simulink model "six_plus_six_AcmsteeringV09_main_1lf"  (R2014a)
settings: Solver=FixedStepDiscrete  StartTime=0.0  StopTime=10.0  FixedStep=0.0005  RelTol=1e-3
InitFcn:
  | Veh_Par_wxt
undefined symbols (not defined in the file or in its folder): acc_spdctl, ag_thr, B, bra_em, bra_pre_gz2, bra_pre_gz34, bra_pre_yd, brakepre_dem_data, brakeTrq_dem_data, bratrq_max, ecucoder_acal, eff_tran, ESP_switch, G, guzhang_lf, guzhang_lm, guzhang_lr, guzhang_rf, guzhang_rm, guzhang_rr, kd1, kd2, ki1, ki2, kp1, kp2, L, myFIS, premax, Radius, RC_switch, s_opt_yi, s_opt_zhuan, s_opt_zhuan_add, s_opt_zhuan_table, spd_map_mot, spd_spdctl, speed_thr_park, TCS_switch, tras_ratio, trq_map_mot, trqmax_yd, trqmax_zx, trqmaxneg, v_gain, v_table, v_thr_park, zhidong_bianmazhi, zhidong_down, zhidong_up, zhidong_youmen, zhuanxiang_bianmazhi, zhuanxiang_down, zhuanxiang_up, zhuanxiang_youmen
libraries: simulink x980, ec5744lib x59, fuzblock x2
(part 3 of 25)

== system six_plus_six_AcmsteeringV09_main_1lf/Data_input/MCU2_1 ==
  In1 : Inport
  In2 : Inport  Port=2
  Trigger : TriggerPort  TriggerType=function-call  PortDimensions=1
  MCU2 : Subsystem
  MCU2_MotorStallingFault : Outport
  MCU2_UdcDetectionFault : Outport  Port=2
  MCU2_TempSensorFault : Outport  Port=3
  MCU2_ActiveDischargingFault : Outport  Port=4
  MCU2_ldcSensorFault : Outport  Port=5
  MCU2_luSensorFault : Outport  Port=6
  MCU2_lvSensorFault : Outport  Port=7
  MCU2_FaultLevel : Outport  Port=8
  MCU2_Controllerload : Outport  Port=9
  MCU2_CanCommunicationFault : Outport  Port=10
  MCU2_MemoryFault : Outport  Port=11
  MCU2_DownratingFault : Outport  Port=12
  MCU2_IGBTFault : Outport  Port=13
  MCU2_MotorOverTemp : Outport  Port=14
  MCU2_ControllerOverTemp : Outport  Port=15
  MCU2_MotorOverSpeed : Outport  Port=16
  MCU2_RotaryInverterFault : Outport  Port=17
  MCU2_UnderVoltage : Outport  Port=18
  MCU2_OverVoltage : Outport  Port=19
  MCU2_MotorOverLoad : Outport  Port=20
  wires:
  MCU2/1(MCU2_MotorStallingFault_Out) -> MCU2_MotorStallingFault/1
  MCU2/7(MCU2_IvSensorFault_Out) -> MCU2_lvSensorFault/1
  MCU2/4(MCU2_ActieDischargingFault_Out) -> MCU2_ActiveDischargingFault/1
  MCU2/12(MCU2_DownratingFault_Out) -> MCU2_DownratingFault/1
  MCU2/13(MCU2_IGBTFault_Out) -> MCU2_IGBTFault/1
  MCU2/3(MCU2_TempSensorFault_Out) -> MCU2_TempSensorFault/1
  MCU2/10(MCU2_CanCommunicationFault_Out) -> MCU2_CanCommunicationFault/1
  MCU2/11(MCU2_MemoryFault_Out) -> MCU2_MemoryFault/1
  MCU2/14(MCU2_MotorOverTemp_Out) -> MCU2_MotorOverTemp/1
  MCU2/2(MCU2_UdcDetectionFault_Out) -> MCU2_UdcDetectionFault/1
  MCU2/5(MCU2_IdcSensorFault_Out) -> MCU2_ldcSensorFault/1
  In2/1 -> MCU2/1(input)
  In1/1 -> MCU2/Enable
  MCU2/6(MCU2_IuSensorFault_Out) -> MCU2_luSensorFault/1
  MCU2/8(MCU2_FaultLevel_Out) -> MCU2_FaultLevel/1
  MCU2/9(MCU2_ControllerOverload_Out) -> MCU2_Controllerload/1
  MCU2/20(MCU2_MotorOverLoad_Out) -> MCU2_MotorOverLoad/1
  MCU2/18(MCU2_UnderVoltage_Out) -> MCU2_UnderVoltage/1
  MCU2/19(MCU2_OverVoltage_Out) -> MCU2_OverVoltage/1
  MCU2/15(MCU2_ControllerOverTemp_Out) -> MCU2_ControllerOverTemp/1
  MCU2/16(MCU2_MotorOverSpeed_Out) -> MCU2_MotorOverSpeed/1
  MCU2/17(MCU2_RotaryInverterFault_Out) -> MCU2_RotaryInverterFault/1

== matlab function six_plus_six_AcmsteeringV09_main_1lf/MainControl/mode_control/backward/backward/Drive/驱动防滑控制TCS/直行TCS/直行/MATLAB Function5 ==
  data: TCS_switch input; flag_lf1 output; flag_lm1 output; flag_lf input; flag_lm input; flag_lr input; flag_lr1 output; flag_rf input; flag_rm input; flag_rr input; flag_rf1 output; flag_rm1 output; flag_rr1 output
 function [flag_lf1,flag_lm1,flag_lr1,flag_rf1,flag_rm1,flag_rr1] = fcn(TCS_switch,flag_lf,flag_lm,flag_lr,flag_rf,flag_rm,flag_rr)
%#codegen
if TCS_switch==0
    flag_lf1=single(0);
    flag_lm1=single(0);
    flag_lr1=single(0);
    flag_rf1=single(0);
    flag_rm1=single(0);
    flag_rr1=single(0);
else
    flag_lf1=single(flag_lf);
    flag_lm1=single(flag_lm);
    flag_lr1=single(flag_lr);
    flag_rf1=single(flag_rf);
    flag_rm1=single(flag_rm);
    flag_rr1=single(flag_rr);
end
end

== matlab function six_plus_six_AcmsteeringV09_main_1lf/Data_input/6/Enabled Subsystem/MATLAB Function1 ==
  data: data1 input; y output; data2 input; data3 input; data4 input
function y = fcn(data1,data2,data3,data4)
%#codegen
y1=data4*256^3+data3*256^2+data2*256+data1;
y=typecast(uint32(y1),'single');
end
% y = u;

== matlab function six_plus_six_AcmsteeringV09_main_1lf/Data_input/10/Enabled Subsystem/MATLAB Function ==
  data: data1 input; y output; data2 input; data3 input; data4 input
function y = fcn(data1,data2,data3,data4)
%#codegen
y1=data4*256^3+data3*256^2+data2*256+data1;
y=typecast(uint32(y1),'single');
end
% y = u;

== matlab function six_plus_six_AcmsteeringV09_main_1lf/MainControl/mode_control/backward/backward/Drive/MATLAB Function ==
  data: acc_y input; y output; ag_thr input
function y = fcn(acc_y,ag_thr)
%#codegen
if abs(acc_y)>=ag_thr
    y=int8(0);
else 
    y=int8(1);
end
end

== system six_plus_six_AcmsteeringV09_main_1lf/Data_input/MCU2_2 ==
  In1 : Inport
  In2 : Inport  Port=2
  Trigger : TriggerPort  TriggerType=function-call  PortDimensions=1
  MCU2 : Subsystem
  MCU2_MotorStallingFault : Outport
  MCU2_UdcDetectionFault : Outport  Port=2
  MCU2_TempSensorFault : Outport  Port=3
  MCU2_ActiveDischargingFault : Outport  Port=4
  MCU2_ldcSensorFault : Outport  Port=5
  MCU2_luSensorFault : Outport  Port=6
  MCU2_lvSensorFault : Outport  Port=7
  MCU2_FaultLevel : Outport  Port=8
  MCU2_Controllerload : Outport  Port=9
  MCU2_CanCommunicationFault : Outport  Port=10
  MCU2_MemoryFault : Outport  Port=11
  MCU2_DownratingFault : Outport  Port=12
  MCU2_IGBTFault : Outport  Port=13
  MCU2_MotorOverTemp : Outport  Port=14
  MCU2_ControllerOverTemp : Outport  Port=15
  MCU2_MotorOverSpeed : Outport  Port=16
  MCU2_RotaryInverterFault : Outport  Port=17
  MCU2_UnderVoltage : Outport  Port=18
  MCU2_OverVoltage : Outport  Port=19
  MCU2_MotorOverLoad : Outport  Port=20
  wires:
  MCU2/1(MCU2_MotorStallingFault_Out) -> MCU2_MotorStallingFault/1
  MCU2/7(MCU2_IvSensorFault_Out) -> MCU2_lvSensorFault/1
  MCU2/4(MCU2_ActieDischargingFault_Out) -> MCU2_ActiveDischargingFault/1
  MCU2/12(MCU2_DownratingFault_Out) -> MCU2_DownratingFault/1
  MCU2/13(MCU2_IGBTFault_Out) -> MCU2_IGBTFault/1
  MCU2/3(MCU2_TempSensorFault_Out) -> MCU2_TempSensorFault/1
  MCU2/10(MCU2_CanCommunicationFault_Out) -> MCU2_CanCommunicationFault/1
  MCU2/11(MCU2_MemoryFault_Out) -> MCU2_MemoryFault/1
  MCU2/14(MCU2_MotorOverTemp_Out) -> MCU2_MotorOverTemp/1
  MCU2/2(MCU2_UdcDetectionFault_Out) -> MCU2_UdcDetectionFault/1
  MCU2/5(MCU2_IdcSensorFault_Out) -> MCU2_ldcSensorFault/1
  In2/1 -> MCU2/1(input)
  In1/1 -> MCU2/Enable
  MCU2/6(MCU2_IuSensorFault_Out) -> MCU2_luSensorFault/1
  MCU2/8(MCU2_FaultLevel_Out) -> MCU2_FaultLevel/1
  MCU2/9(MCU2_ControllerOverload_Out) -> MCU2_Controllerload/1
  MCU2/20(MCU2_MotorOverLoad_Out) -> MCU2_MotorOverLoad/1
  MCU2/18(MCU2_UnderVoltage_Out) -> MCU2_UnderVoltage/1
  MCU2/19(MCU2_OverVoltage_Out) -> MCU2_OverVoltage/1
  MCU2/15(MCU2_ControllerOverTemp_Out) -> MCU2_ControllerOverTemp/1
  MCU2/16(MCU2_MotorOverSpeed_Out) -> MCU2_MotorOverSpeed/1
  MCU2/17(MCU2_RotaryInverterFault_Out) -> MCU2_RotaryInverterFault/1

== system six_plus_six_AcmsteeringV09_main_1lf/Data_input/MCU2_3 ==
  In1 : Inport
  In2 : Inport  Port=2
  Trigger : TriggerPort  TriggerType=function-call  PortDimensions=1
  MCU2 : Subsystem
  MCU2_MotorStallingFault : Outport
  MCU2_UdcDetectionFault : Outport  Port=2
  MCU2_TempSensorFault : Outport  Port=3
  MCU2_ActiveDischargingFault : Outport  Port=4
  MCU2_ldcSensorFault : Outport  Port=5
  MCU2_luSensorFault : Outport  Port=6
  MCU2_lvSensorFault : Outport  Port=7
  MCU2_FaultLevel : Outport  Port=8
  MCU2_Controllerload : Outport  Port=9
  MCU2_CanCommunicationFault : Outport  Port=10
  MCU2_MemoryFault : Outport  Port=11
  MCU2_DownratingFault : Outport  Port=12
  MCU2_IGBTFault : Outport  Port=13
  MCU2_MotorOverTemp : Outport  Port=14
  MCU2_ControllerOverTemp : Outport  Port=15
  MCU2_MotorOverSpeed : Outport  Port=16
  MCU2_RotaryInverterFault : Outport  Port=17
  MCU2_UnderVoltage : Outport  Port=18
  MCU2_OverVoltage : Outport  Port=19
  MCU2_MotorOverLoad : Outport  Port=20
  wires:
  MCU2/1(MCU2_MotorStallingFault_Out) -> MCU2_MotorStallingFault/1
  MCU2/7(MCU2_IvSensorFault_Out) -> MCU2_lvSensorFault/1
  MCU2/4(MCU2_ActieDischargingFault_Out) -> MCU2_ActiveDischargingFault/1
  MCU2/12(MCU2_DownratingFault_Out) -> MCU2_DownratingFault/1
  MCU2/13(MCU2_IGBTFault_Out) -> MCU2_IGBTFault/1
  MCU2/3(MCU2_TempSensorFault_Out) -> MCU2_TempSensorFault/1
  MCU2/10(MCU2_CanCommunicationFault_Out) -> MCU2_CanCommunicationFault/1
  MCU2/11(MCU2_MemoryFault_Out) -> MCU2_MemoryFault/1
  MCU2/14(MCU2_MotorOverTemp_Out) -> MCU2_MotorOverTemp/1
  MCU2/2(MCU2_UdcDetectionFault_Out) -> MCU2_UdcDetectionFault/1
  MCU2/5(MCU2_IdcSensorFault_Out) -> MCU2_ldcSensorFault/1
  In2/1 -> MCU2/1(input)
  In1/1 -> MCU2/Enable
  MCU2/6(MCU2_IuSensorFault_Out) -> MCU2_luSensorFault/1
  MCU2/8(MCU2_FaultLevel_Out) -> MCU2_FaultLevel/1
  MCU2/9(MCU2_ControllerOverload_Out) -> MCU2_Controllerload/1
  MCU2/20(MCU2_MotorOverLoad_Out) -> MCU2_MotorOverLoad/1
  MCU2/18(MCU2_UnderVoltage_Out) -> MCU2_UnderVoltage/1
  MCU2/19(MCU2_OverVoltage_Out) -> MCU2_OverVoltage/1
  MCU2/15(MCU2_ControllerOverTemp_Out) -> MCU2_ControllerOverTemp/1
  MCU2/16(MCU2_MotorOverSpeed_Out) -> MCU2_MotorOverSpeed/1
  MCU2/17(MCU2_RotaryInverterFault_Out) -> MCU2_RotaryInverterFault/1

== system six_plus_six_AcmsteeringV09_main_1lf/Data_input/MCU2_4 ==
  In1 : Inport
  In2 : Inport  Port=2
  Trigger : TriggerPort  TriggerType=function-call  PortDimensions=1
  MCU2 : Subsystem
  MCU2_MotorStallingFault : Outport
  MCU2_UdcDetectionFault : Outport  Port=2
  MCU2_TempSensorFault : Outport  Port=3
  MCU2_ActiveDischargingFault : Outport  Port=4
  MCU2_ldcSensorFault : Outport  Port=5
  MCU2_luSensorFault : Outport  Port=6
  MCU2_lvSensorFault : Outport  Port=7
  MCU2_FaultLevel : Outport  Port=8
  MCU2_Controllerload : Outport  Port=9
  MCU2_CanCommunicationFault : Outport  Port=10
  MCU2_MemoryFault : Outport  Port=11
  MCU2_DownratingFault : Outport  Port=12
  MCU2_IGBTFault : Outport  Port=13
  MCU2_MotorOverTemp : Outport  Port=14
  MCU2_ControllerOverTemp : Outport  Port=15
  MCU2_MotorOverSpeed : Outport  Port=16
  MCU2_RotaryInverterFault : Outport  Port=17
  MCU2_UnderVoltage : Outport  Port=18
  MCU2_OverVoltage : Outport  Port=19
  MCU2_MotorOverLoad : Outport  Port=20
  wires:
  MCU2/1(MCU2_MotorStallingFault_Out) -> MCU2_MotorStallingFault/1
  MCU2/7(MCU2_IvSensorFault_Out) -> MCU2_lvSensorFault/1
  MCU2/4(MCU2_ActieDischargingFault_Out) -> MCU2_ActiveDischargingFault/1
  MCU2/12(MCU2_DownratingFault_Out) -> MCU2_DownratingFault/1
  MCU2/13(MCU2_IGBTFault_Out) -> MCU2_IGBTFault/1
  MCU2/3(MCU2_TempSensorFault_Out) -> MCU2_TempSensorFault/1
  MCU2/10(MCU2_CanCommunicationFault_Out) -> MCU2_CanCommunicationFault/1
  MCU2/11(MCU2_MemoryFault_Out) -> MCU2_MemoryFault/1
  MCU2/14(MCU2_MotorOverTemp_Out) -> MCU2_MotorOverTemp/1
  MCU2/2(MCU2_UdcDetectionFault_Out) -> MCU2_UdcDetectionFault/1
  MCU2/5(MCU2_IdcSensorFault_Out) -> MCU2_ldcSensorFault/1
  In2/1 -> MCU2/1(input)
  In1/1 -> MCU2/Enable
  MCU2/6(MCU2_IuSensorFault_Out) -> MCU2_luSensorFault/1
  MCU2/8(MCU2_FaultLevel_Out) -> MCU2_FaultLevel/1
  MCU2/9(MCU2_ControllerOverload_Out) -> MCU2_Controllerload/1
  MCU2/20(MCU2_MotorOverLoad_Out) -> MCU2_MotorOverLoad/1
  MCU2/18(MCU2_UnderVoltage_Out) -> MCU2_UnderVoltage/1
  MCU2/19(MCU2_OverVoltage_Out) -> MCU2_OverVoltage/1
  MCU2/15(MCU2_ControllerOverTemp_Out) -> MCU2_ControllerOverTemp/1
  MCU2/16(MCU2_MotorOverSpeed_Out) -> MCU2_MotorOverSpeed/1
  MCU2/17(MCU2_RotaryInverterFault_Out) -> MCU2_RotaryInverterFault/1

== system six_plus_six_AcmsteeringV09_main_1lf/Data_input/MCU2_5 ==
  In1 : Inport
  In2 : Inport  Port=2
  Trigger : TriggerPort  TriggerType=function-call  PortDimensions=1
  MCU2 : Subsystem
  MCU2_MotorStallingFault : Outport
  MCU2_UdcDetectionFault : Outport  Port=2
  MCU2_TempSensorFault : Outport  Port=3
  MCU2_ActiveDischargingFault : Outport  Port=4
  MCU2_ldcSensorFault : Outport  Port=5
  MCU2_luSensorFault : Outport  Port=6
  MCU2_lvSensorFault : Outport  Port=7
  MCU2_FaultLevel : Outport  Port=8
  MCU2_Controllerload : Outport  Port=9
  MCU2_CanCommunicationFault : Outport  Port=10
  MCU2_MemoryFault : Outport  Port=11
  MCU2_DownratingFault : Outport  Port=12
  MCU2_IGBTFault : Outport  Port=13
  MCU2_MotorOverTemp : Outport  Port=14
  MCU2_ControllerOverTemp : Outport  Port=15
  MCU2_MotorOverSpeed : Outport  Port=16
  MCU2_RotaryInverterFault : Outport  Port=17
  MCU2_UnderVoltage : Outport  Port=18
  MCU2_OverVoltage : Outport  Port=19
  MCU2_MotorOverLoad : Outport  Port=20
  wires:
  MCU2/1(MCU2_MotorStallingFault_Out) -> MCU2_MotorStallingFault/1
  MCU2/7(MCU2_IvSensorFault_Out) -> MCU2_lvSensorFault/1
  MCU2/4(MCU2_ActieDischargingFault_Out) -> MCU2_ActiveDischargingFault/1
  MCU2/12(MCU2_DownratingFault_Out) -> MCU2_DownratingFault/1
  MCU2/13(MCU2_IGBTFault_Out) -> MCU2_IGBTFault/1
  MCU2/3(MCU2_TempSensorFault_Out) -> MCU2_TempSensorFault/1
  MCU2/10(MCU2_CanCommunicationFault_Out) -> MCU2_CanCommunicationFault/1
  MCU2/11(MCU2_MemoryFault_Out) -> MCU2_MemoryFault/1
  MCU2/14(MCU2_MotorOverTemp_Out) -> MCU2_MotorOverTemp/1
  MCU2/2(MCU2_UdcDetectionFault_Out) -> MCU2_UdcDetectionFault/1
  MCU2/5(MCU2_IdcSensorFault_Out) -> MCU2_ldcSensorFault/1
  In2/1 -> MCU2/1(input)
  In1/1 -> MCU2/Enable
  MCU2/6(MCU2_IuSensorFault_Out) -> MCU2_luSensorFault/1
  MCU2/8(MCU2_FaultLevel_Out) -> MCU2_FaultLevel/1
  MCU2/9(MCU2_ControllerOverload_Out) -> MCU2_Controllerload/1
  MCU2/20(MCU2_MotorOverLoad_Out) -> MCU2_MotorOverLoad/1
  MCU2/18(MCU2_UnderVoltage_Out) -> MCU2_UnderVoltage/1
  MCU2/19(MCU2_OverVoltage_Out) -> MCU2_OverVoltage/1
  MCU2/15(MCU2_ControllerOverTemp_Out) -> MCU2_ControllerOverTemp/1
  MCU2/16(MCU2_MotorOverSpeed_Out) -> MCU2_MotorOverSpeed/1
  MCU2/17(MCU2_RotaryInverterFault_Out) -> MCU2_RotaryInverterFault/1

== system six_plus_six_AcmsteeringV09_main_1lf/Data_input/RemoteControl1 ==
  In1 : Inport
  In2 : Inport  Port=2
  Trigger : TriggerPort  TriggerType=function-call  PortDimensions=1
  Yaokong2 : Subsystem
  SH : Outport
  SE : Outport  Port=2
  SD : Outport  Port=3
  SA : Outport  Port=4
  LIFEspan : Outport  Port=5
  wires:
  Yaokong2/2(SE_Out) -> SE/1
  Yaokong2/3(SD_Out) -> SD/1
  Yaokong2/4(SA_Out) -> SA/1
  In2/1 -> Yaokong2/1(input)
  In1/1 -> Yaokong2/Enable
  Yaokong2/1(SH_Out) -> SH/1
  Yaokong2/5(LIFEspan_Out) -> LIFEspan/1

== system six_plus_six_AcmsteeringV09_main_1lf/Data_input/RemoteControl2 ==
  In1 : Inport
  In2 : Inport  Port=2
  Trigger : TriggerPort  TriggerType=function-call  PortDimensions=1
  Yaokong1 : Subsystem
  Rightstick_updown : Outport
  Rightstick_leftright : Outport  Port=2
  Leftstick_updown : Outport  Port=3
  Leftstick_leftright : Outport  Port=4
  wires:
  In1/1 -> Yaokong1/Enable
  In2/1 -> Yaokong1/1(input)
  Yaokong1/1(Rightstick_updown_Out) -> Rightstick_updown/1
  Yaokong1/2(Rightstick_leftright_Out) -> Rightstick_leftright/1
  Yaokong1/3(Leftstick_updown_Out) -> Leftstick_updown/1
  Yaokong1/4(Leftstick_leftright_Out) -> Leftstick_leftright/1

== system six_plus_six_AcmsteeringV09_main_1lf/MainControl/mode_control ==
  mode_dem_out : Inport
  Signals : Inport  Port=2
  Multiport Switch : MultiPortSwitch  DataPortOrder=Zero-based contiguous  Inputs=6
  Park : Subsystem  TreatAsAtomicUnit=on
  Switch Case : SwitchCase  CaseConditions={0,1,2,3,4,5}  ShowDefaultCase=off
  backward : Subsystem  TreatAsAtomicUnit=on
  center_steer : Subsystem  TreatAsAtomicUnit=on
  emergency_stop : Subsystem  TreatAsAtomicUnit=on
  forward : Subsystem  TreatAsAtomicUnit=on
  neutral : Subsystem  TreatAsAtomicUnit=on
  com_dem : Outport
  wires:
  mode_dem_out/1 -> Multiport Switch/1, Switch Case/1
  Signals/1 -> backward/1(Signals), emergency_stop/1(Signals), center_steer/1(Signals), neutral/1(Signals), forward/1(Signals), Park/1(Signals)
  Switch Case/1 -> Park/Action
  Switch Case/6 -> emergency_stop/Action
  Switch Case/5 -> center_steer/Action
  Switch Case/4 -> backward/Action
  Switch Case/3 -> neutral/Action
  Switch Case/2 -> forward/Action
  Park/1(park_dem) -> Multiport Switch/2
  forward/1(forward_dem) -> Multiport Switch/3
  backward/1(backward_dem) -> Multiport Switch/5
  neutral/1(neutral_dem) -> Multiport Switch/4
  center_steer/1(center_steer_dem) -> Multiport Switch/6
  emergency_stop/1(emergency_stop_dem) -> Multiport Switch/7
  Multiport Switch/1 -> com_dem/1

== system six_plus_six_AcmsteeringV09_main_1lf/MainControl/mode_switch ==
  Signals : Inport
  Abs{,1..5} (6 alike) : Abs  OutDataTypeStr=single
  Bus Selector : BusSelector  OutputSignals=RemoteControl_dem.brake_emerg,RemoteControl_dem.park,RemoteControl_dem.acc_dem,RemoteControl_dem.steer_dem,RemoteControl_dem.brake_dem,RemoteControl_dem.center,MOTOR.MOTOR1.MCU0.MCU0_SpeedFdk,MOTOR.MOTOR2.MCU0_1.MCU0_1SpeedFdk,MOTOR.MOTOR3.MCU0_2.MCU0_2SpeedFdk,MOTOR.MOTOR4.MCU0_3.MCU0_3SpeedFdk,MOTOR.MOTOR5.MCU0_4.MCU0_4SpeedFdk,MOTOR.MOTOR6.MCU0_5.MCU0_5SpeedFdk
  Constant1 : Constant  Value=v_thr_park  OutDataTypeStr=single  SampleTime=-1
  Constant2 : Constant  Value=speed_thr_park  OutDataTypeStr=single  SampleTime=-1
  Memory : Memory  InheritSampleTime=on
  Terminator : Terminator
  mode_switch : MATLAB Function  TreatAsAtomicUnit=on
  mode_dem_out : Outport
  wires:
  Memory/1 -> mode_switch/14(mode_dem_out_pre)
  Signals/1 -> Bus Selector/1
  Constant2/1 -> mode_switch/13(speed_thr_park)
  mode_switch/1(mode_dem_out) -> Memory/1, mode_dem_out/1  "mode_dem_out"
  Bus Selector/1 -> mode_switch/1(brake_emerg)  "<brake_emerg>"
  Bus Selector/2 -> mode_switch/2(park)  "<park>"
  Bus Selector/3 -> mode_switch/3(acc_dem)  "<acc_dem>"
  Bus Selector/4 -> mode_switch/4(steer_dem)  "<steer_dem>"
  Bus Selector/5 -> mode_switch/5(brake_dem)  "<brake_dem>"
  Bus Selector/7 -> Abs/1  "<MCU0_SpeedFdk>"
  Bus Selector/8 -> Abs1/1  "<MCU0_1SpeedFdk>"
  Bus Selector/9 -> Abs2/1  "<MCU0_2SpeedFdk>"
  Bus Selector/10 -> Abs3/1  "<MCU0_3SpeedFdk>"
  Bus Selector/11 -> Abs4/1  "<MCU0_4SpeedFdk>"
  Bus Selector/12 -> Abs5/1  "<MCU0_5SpeedFdk>"
  Abs/1 -> mode_switch/7(MCU0_SpeedFdk)
  Abs1/1 -> mode_switch/8(MCU0_1SpeedFdk)
  Abs2/1 -> mode_switch/9(MCU0_2SpeedFdk)
  Abs3/1 -> mode_switch/10(MCU0_3SpeedFdk)
  Abs4/1 -> mode_switch/11(MCU0_4SpeedFdk)
  Abs5/1 -> mode_switch/12(MCU0_5SpeedFdk)
  Constant1/1 -> Terminator/1
  Bus Selector/6 -> mode_switch/6(center)  "<center>"

== system six_plus_six_AcmsteeringV09_main_1lf/Subsystem/VCU1 ==
  VCU1_EnableReq_in : Inport
  VCU1_CtrlModel_in : Inport  Port=2
  VCU1_GearCmd_in : Inport  Port=3
  VCU1_SpeedMax_in : Inport  Port=4
  VCU1_TorqueRef_in : Inport  Port=5
  VCU1_LifeCnt_in : Inport  Port=6
  Conv{1..8} (8 alike) : DataTypeConversion
  VCU1_CtrlModel : Subsystem
  VCU1_DLC : Constant  Value=8  OutDataTypeStr=uint8
  VCU1_DLC_Out : Terminator
  VCU1_EnableReq : Subsystem
  VCU1_GearCmd : Subsystem
  VCU1_ID : Constant  Value=2353065767  OutDataTypeStr=single
  VCU1_ID_Out : Terminator
  VCU1_LifeCnt : Subsystem
  VCU1_SpeedMax : Subsystem
  VCU1_TorqueRef : Subsystem
  VCU1_mux : Mux  Inputs=8
  or{1..8} (8 alike) : simulink/Logic and Bit Operations/Bitwise Operator  logicop=OR  UseBitMask=off  NumInputPorts=6  BitMask=bin2dec('11011001')  BitMaskRealWorld=Stored Integer
  output : Outport
  wires:
  VCU1_mux/1 -> output/1
  VCU1_LifeCnt/1(output1) -> or1/1
  VCU1_LifeCnt/2(output2) -> or2/1
  VCU1_LifeCnt/3(output3) -> or3/1
  VCU1_LifeCnt/4(output4) -> or4/1
  VCU1_LifeCnt/5(output5) -> or5/1
  VCU1_LifeCnt/6(output6) -> or6/1
  VCU1_LifeCnt/7(output7) -> or7/1
  VCU1_LifeCnt/8(output8) -> or8/1
  VCU1_TorqueRef/1(output1) -> or1/2
  VCU1_TorqueRef/2(output2) -> or2/2
  VCU1_TorqueRef/3(output3) -> or3/2
  VCU1_TorqueRef/4(output4) -> or4/2
  VCU1_TorqueRef/5(output5) -> or5/2
  VCU1_TorqueRef/6(output6) -> or6/2
  VCU1_TorqueRef/7(output7) -> or7/2
  VCU1_TorqueRef/8(output8) -> or8/2
  VCU1_SpeedMax/1(output1) -> or1/3
  VCU1_SpeedMax/2(output2) -> or2/3
  VCU1_SpeedMax/3(output3) -> or3/3
  VCU1_SpeedMax/4(output4) -> or4/3
  VCU1_SpeedMax/5(output5) -> or5/3
  VCU1_SpeedMax/6(output6) -> or6/3
  VCU1_SpeedMax/7(output7) -> or7/3
  VCU1_SpeedMax/8(output8) -> or8/3
  VCU1_GearCmd/1(output1) -> or1/4
  VCU1_GearCmd/2(output2) -> or2/4
  VCU1_GearCmd/3(output3) -> or3/4
  VCU1_GearCmd/4(output4) -> or4/4
  VCU1_GearCmd/5(output5) -> or5/4
  VCU1_GearCmd/6(output6) -> or6/4
  VCU1_GearCmd/7(output7) -> or7/4
  VCU1_GearCmd/8(output8) -> or8/4
  VCU1_CtrlModel/1(output1) -> or1/5
  VCU1_CtrlModel/2(output2) -> or2/5
  VCU1_CtrlModel/3(output3) -> or3/5
  VCU1_CtrlModel/4(output4) -> or4/5
  VCU1_CtrlModel/5(output5) -> or5/5
  VCU1_CtrlModel/6(output6) -> or6/5
  VCU1_CtrlModel/7(output7) -> or7/5
  VCU1_CtrlModel/8(output8) -> or8/5
  VCU1_EnableReq/1(output1) -> or1/6
  VCU1_EnableReq/2(output2) -> or2/6
  VCU1_EnableReq/3(output3) -> or3/6
  VCU1_EnableReq/4(output4) -> or4/6
  VCU1_EnableReq/5(output5) -> or5/6
  VCU1_EnableReq/6(output6) -> or6/6
  VCU1_EnableReq/7(output7) -> or7/6
  VCU1_EnableReq/8(output8) -> or8/6
  or1/1 -> Conv1/1
  Conv1/1 -> VCU1_mux/1
  or2/1 -> Conv2/1
  Conv2/1 -> VCU1_mux/2
  or3/1 -> Conv3/1
  Conv3/1 -> VCU1_mux/3
  or4/1 -> Conv4/1
  Conv4/1 -> VCU1_mux/4
  or5/1 -> Conv5/1
  Conv5/1 -> VCU1_mux/5
  or6/1 -> Conv6/1
  Conv6/1 -> VCU1_mux/6
  or7/1 -> Conv7/1
  Conv7/1 -> VCU1_mux/7
  or8/1 -> Conv8/1
  Conv8/1 -> VCU1_mux/8
  VCU1_ID/1 -> VCU1_ID_Out/1
  VCU1_DLC/1 -> VCU1_DLC_Out/1
  VCU1_LifeCnt_in/1 -> VCU1_LifeCnt/1(VCU1_LifeCnt)
  VCU1_TorqueRef_in/1 -> VCU1_TorqueRef/1(VCU1_TorqueRef)
  VCU1_SpeedMax_in/1 -> VCU1_SpeedMax/1(VCU1_SpeedMax)
  VCU1_GearCmd_in/1 -> VCU1_GearCmd/1(VCU1_GearCmd)
  VCU1_CtrlModel_in/1 -> VCU1_CtrlModel/1(VCU1_CtrlModel)
  VCU1_EnableReq_in/1 -> VCU1_EnableReq/1(VCU1_EnableReq)

== system six_plus_six_AcmsteeringV09_main_1lf/Subsystem/VCU2 ==
  VCU1_EnableReq_in : Inport
  VCU1_CtrlModel_in : Inport  Port=2
  VCU1_GearCmd_in : Inport  Port=3
  VCU1_SpeedMax_in : Inport  Port=4
  VCU1_TorqueRef_in : Inport  Port=5
  VCU1_LifeCnt_in : Inport  Port=6
  Conv{1..8} (8 alike) : DataTypeConversion
  VCU1_CtrlModel : Subsystem
  VCU1_DLC : Constant  Value=8  OutDataTypeStr=uint8
  VCU1_DLC_Out : Terminator
  VCU1_EnableReq : Subsystem
  VCU1_GearCmd : Subsystem
  VCU1_ID : Constant  Value=2353065767  OutDataTypeStr=single
  VCU1_ID_Out : Terminator
  VCU1_LifeCnt : Subsystem
  VCU1_SpeedMax : Subsystem
  VCU1_TorqueRef : Subsystem
  VCU1_mux : Mux  Inputs=8
  or{1..8} (8 alike) : simulink/Logic and Bit Operations/Bitwise Operator  logicop=OR  UseBitMask=off  NumInputPorts=6  BitMask=bin2dec('11011001')  BitMaskRealWorld=Stored Integer
  output : Outport
  wires:
  VCU1_mux/1 -> output/1
  VCU1_LifeCnt/1(output1) -> or1/1
  VCU1_LifeCnt/2(output2) -> or2/1
  VCU1_LifeCnt/3(output3) -> or3/1
  VCU1_LifeCnt/4(output4) -> or4/1
  VCU1_LifeCnt/5(output5) -> or5/1
  VCU1_LifeCnt/6(output6) -> or6/1
  VCU1_LifeCnt/7(output7) -> or7/1
  VCU1_LifeCnt/8(output8) -> or8/1
  VCU1_TorqueRef/1(output1) -> or1/2
  VCU1_TorqueRef/2(output2) -> or2/2
  VCU1_TorqueRef/3(output3) -> or3/2
  VCU1_TorqueRef/4(output4) -> or4/2
  VCU1_TorqueRef/5(output5) -> or5/2
  VCU1_TorqueRef/6(output6) -> or6/2
  VCU1_TorqueRef/7(output7) -> or7/2
  VCU1_TorqueRef/8(output8) -> or8/2
  VCU1_SpeedMax/1(output1) -> or1/3
  VCU1_SpeedMax/2(output2) -> or2/3
  VCU1_SpeedMax/3(output3) -> or3/3
  VCU1_SpeedMax/4(output4) -> or4/3
  VCU1_SpeedMax/5(output5) -> or5/3
  VCU1_SpeedMax/6(output6) -> or6/3
  VCU1_SpeedMax/7(output7) -> or7/3
  VCU1_SpeedMax/8(output8) -> or8/3
  VCU1_GearCmd/1(output1) -> or1/4
  VCU1_GearCmd/2(output2) -> or2/4
  VCU1_GearCmd/3(output3) -> or3/4
  VCU1_GearCmd/4(output4) -> or4/4
  VCU1_GearCmd/5(output5) -> or5/4
  VCU1_GearCmd/6(output6) -> or6/4
  VCU1_GearCmd/7(output7) -> or7/4
  VCU1_GearCmd/8(output8) -> or8/4
  VCU1_CtrlModel/1(output1) -> or1/5
  VCU1_CtrlModel/2(output2) -> or2/5
  VCU1_CtrlModel/3(output3) -> or3/5
  VCU1_CtrlModel/4(output4) -> or4/5
  VCU1_CtrlModel/5(output5) -> or5/5
  VCU1_CtrlModel/6(output6) -> or6/5
  VCU1_CtrlModel/7(output7) -> or7/5
  VCU1_CtrlModel/8(output8) -> or8/5
  VCU1_EnableReq/1(output1) -> or1/6
  VCU1_EnableReq/2(output2) -> or2/6
  VCU1_EnableReq/3(output3) -> or3/6
  VCU1_EnableReq/4(output4) -> or4/6
  VCU1_EnableReq/5(output5) -> or5/6
  VCU1_EnableReq/6(output6) -> or6/6
  VCU1_EnableReq/7(output7) -> or7/6
  VCU1_EnableReq/8(output8) -> or8/6
  or1/1 -> Conv1/1
  Conv1/1 -> VCU1_mux/1
  or2/1 -> Conv2/1
  Conv2/1 -> VCU1_mux/2
  or3/1 -> Conv3/1
  Conv3/1 -> VCU1_mux/3
  or4/1 -> Conv4/1
  Conv4/1 -> VCU1_mux/4
  or5/1 -> Conv5/1
  Conv5/1 -> VCU1_mux/5
  or6/1 -> Conv6/1
  Conv6/1 -> VCU1_mux/6
  or7/1 -> Conv7/1
  Conv7/1 -> VCU1_mux/7
  or8/1 -> Conv8/1
  Conv8/1 -> VCU1_mux/8
  VCU1_ID/1 -> VCU1_ID_Out/1
  VCU1_DLC/1 -> VCU1_DLC_Out/1
  VCU1_LifeCnt_in/1 -> VCU1_LifeCnt/1(VCU1_LifeCnt)
  VCU1_TorqueRef_in/1 -> VCU1_TorqueRef/1(VCU1_TorqueRef)
  VCU1_SpeedMax_in/1 -> VCU1_SpeedMax/1(VCU1_SpeedMax)
  VCU1_GearCmd_in/1 -> VCU1_GearCmd/1(VCU1_GearCmd)
  VCU1_CtrlModel_in/1 -> VCU1_CtrlModel/1(VCU1_CtrlModel)
  VCU1_EnableReq_in/1 -> VCU1_EnableReq/1(VCU1_EnableReq)

== system six_plus_six_AcmsteeringV09_main_1lf/Subsystem/VCU3 ==
  VCU1_EnableReq_in : Inport
  VCU1_CtrlModel_in : Inport  Port=2
  VCU1_GearCmd_in : Inport  Port=3
  VCU1_SpeedMax_in : Inport  Port=4
  VCU1_TorqueRef_in : Inport  Port=5
  VCU1_LifeCnt_in : Inport  Port=6
  Conv{1..8} (8 alike) : DataTypeConversion
  VCU1_CtrlModel : Subsystem
  VCU1_DLC : Constant  Value=8  OutDataTypeStr=uint8
  VCU1_DLC_Out : Terminator
  VCU1_EnableReq : Subsystem
  VCU1_GearCmd : Subsystem
  VCU1_ID : Constant  Value=2353065767  OutDataTypeStr=single
  VCU1_ID_Out : Terminator
  VCU1_LifeCnt : Subsystem
  VCU1_SpeedMax : Subsystem
  VCU1_TorqueRef : Subsystem
  VCU1_mux : Mux  Inputs=8
  or{1..8} (8 alike) : simulink/Logic and Bit Operations/Bitwise Operator  logicop=OR  UseBitMask=off  NumInputPorts=6  BitMask=bin2dec('11011001')  BitMaskRealWorld=Stored Integer
  output : Outport
  wires:
  VCU1_mux/1 -> output/1
  VCU1_LifeCnt/1(output1) -> or1/1
  VCU1_LifeCnt/2(output2) -> or2/1
  VCU1_LifeCnt/3(output3) -> or3/1
  VCU1_LifeCnt/4(output4) -> or4/1
  VCU1_LifeCnt/5(output5) -> or5/1
  VCU1_LifeCnt/6(output6) -> or6/1
  VCU1_LifeCnt/7(output7) -> or7/1
  VCU1_LifeCnt/8(output8) -> or8/1
  VCU1_TorqueRef/1(output1) -> or1/2
  VCU1_TorqueRef/2(output2) -> or2/2
  VCU1_TorqueRef/3(output3) -> or3/2
  VCU1_TorqueRef/4(output4) -> or4/2
  VCU1_TorqueRef/5(output5) -> or5/2
  VCU1_TorqueRef/6(output6) -> or6/2
  VCU1_TorqueRef/7(output7) -> or7/2
  VCU1_TorqueRef/8(output8) -> or8/2
  VCU1_SpeedMax/1(output1) -> or1/3
  VCU1_SpeedMax/2(output2) -> or2/3
  VCU1_SpeedMax/3(output3) -> or3/3
  VCU1_SpeedMax/4(output4) -> or4/3
  VCU1_SpeedMax/5(output5) -> or5/3
  VCU1_SpeedMax/6(output6) -> or6/3
  VCU1_SpeedMax/7(output7) -> or7/3
  VCU1_SpeedMax/8(output8) -> or8/3
  VCU1_GearCmd/1(output1) -> or1/4
  VCU1_GearCmd/2(output2) -> or2/4
  VCU1_GearCmd/3(output3) -> or3/4
  VCU1_GearCmd/4(output4) -> or4/4
  VCU1_GearCmd/5(output5) -> or5/4
  VCU1_GearCmd/6(output6) -> or6/4
  VCU1_GearCmd/7(output7) -> or7/4
  VCU1_GearCmd/8(output8) -> or8/4
  VCU1_CtrlModel/1(output1) -> or1/5
  VCU1_CtrlModel/2(output2) -> or2/5
  VCU1_CtrlModel/3(output3) -> or3/5
  VCU1_CtrlModel/4(output4) -> or4/5
  VCU1_CtrlModel/5(output5) -> or5/5
  VCU1_CtrlModel/6(output6) -> or6/5
  VCU1_CtrlModel/7(output7) -> or7/5
  VCU1_CtrlModel/8(output8) -> or8/5
  VCU1_EnableReq/1(output1) -> or1/6
  VCU1_EnableReq/2(output2) -> or2/6
  VCU1_EnableReq/3(output3) -> or3/6
  VCU1_EnableReq/4(output4) -> or4/6
  VCU1_EnableReq/5(output5) -> or5/6
  VCU1_EnableReq/6(output6) -> or6/6
  VCU1_EnableReq/7(output7) -> or7/6
  VCU1_EnableReq/8(output8) -> or8/6
  or1/1 -> Conv1/1
  Conv1/1 -> VCU1_mux/1
  or2/1 -> Conv2/1
  Conv2/1 -> VCU1_mux/2
  or3/1 -> Conv3/1
  Conv3/1 -> VCU1_mux/3
  or4/1 -> Conv4/1
  Conv4/1 -> VCU1_mux/4
  or5/1 -> Conv5/1
  Conv5/1 -> VCU1_mux/5
  or6/1 -> Conv6/1
  Conv6/1 -> VCU1_mux/6
  or7/1 -> Conv7/1
  Conv7/1 -> VCU1_mux/7
  or8/1 -> Conv8/1
  Conv8/1 -> VCU1_mux/8
  VCU1_ID/1 -> VCU1_ID_Out/1
  VCU1_DLC/1 -> VCU1_DLC_Out/1
  VCU1_LifeCnt_in/1 -> VCU1_LifeCnt/1(VCU1_LifeCnt)
  VCU1_TorqueRef_in/1 -> VCU1_TorqueRef/1(VCU1_TorqueRef)
  VCU1_SpeedMax_in/1 -> VCU1_SpeedMax/1(VCU1_SpeedMax)
  VCU1_GearCmd_in/1 -> VCU1_GearCmd/1(VCU1_GearCmd)
  VCU1_CtrlModel_in/1 -> VCU1_CtrlModel/1(VCU1_CtrlModel)
  VCU1_EnableReq_in/1 -> VCU1_EnableReq/1(VCU1_EnableReq)

== system six_plus_six_AcmsteeringV09_main_1lf/Subsystem/VCU4 ==
  VCU1_EnableReq_in : Inport
  VCU1_CtrlModel_in : Inport  Port=2
  VCU1_GearCmd_in : Inport  Port=3
  VCU1_SpeedMax_in : Inport  Port=4
  VCU1_TorqueRef_in : Inport  Port=5
  VCU1_LifeCnt_in : Inport  Port=6
  Conv{1..8} (8 alike) : DataTypeConversion
  VCU1_CtrlModel : Subsystem
  VCU1_DLC : Constant  Value=8  OutDataTypeStr=uint8
  VCU1_DLC_Out : Terminator
  VCU1_EnableReq : Subsystem
  VCU1_GearCmd : Subsystem
  VCU1_ID : Constant  Value=2353065767  OutDataTypeStr=single
  VCU1_ID_Out : Terminator
  VCU1_LifeCnt : Subsystem
  VCU1_SpeedMax : Subsystem
  VCU1_TorqueRef : Subsystem
  VCU1_mux : Mux  Inputs=8
  or{1..8} (8 alike) : simulink/Logic and Bit Operations/Bitwise Operator  logicop=OR  UseBitMask=off  NumInputPorts=6  BitMask=bin2dec('11011001')  BitMaskRealWorld=Stored Integer
  output : Outport
  wires:
  VCU1_mux/1 -> output/1
  VCU1_LifeCnt/1(output1) -> or1/1
  VCU1_LifeCnt/2(output2) -> or2/1
  VCU1_LifeCnt/3(output3) -> or3/1
  VCU1_LifeCnt/4(output4) -> or4/1
  VCU1_LifeCnt/5(output5) -> or5/1
  VCU1_LifeCnt/6(output6) -> or6/1
  VCU1_LifeCnt/7(output7) -> or7/1
  VCU1_LifeCnt/8(output8) -> or8/1
  VCU1_TorqueRef/1(output1) -> or1/2
  VCU1_TorqueRef/2(output2) -> or2/2
  VCU1_TorqueRef/3(output3) -> or3/2
  VCU1_TorqueRef/4(output4) -> or4/2
  VCU1_TorqueRef/5(output5) -> or5/2
  VCU1_TorqueRef/6(output6) -> or6/2
  VCU1_TorqueRef/7(output7) -> or7/2
  VCU1_TorqueRef/8(output8) -> or8/2
  VCU1_SpeedMax/1(output1) -> or1/3
  VCU1_SpeedMax/2(output2) -> or2/3
  VCU1_SpeedMax/3(output3) -> or3/3
  VCU1_SpeedMax/4(output4) -> or4/3
  VCU1_SpeedMax/5(output5) -> or5/3
  VCU1_SpeedMax/6(output6) -> or6/3
  VCU1_SpeedMax/7(output7) -> or7/3
  VCU1_SpeedMax/8(output8) -> or8/3
  VCU1_GearCmd/1(output1) -> or1/4
  VCU1_GearCmd/2(output2) -> or2/4
  VCU1_GearCmd/3(output3) -> or3/4
  VCU1_GearCmd/4(output4) -> or4/4
  VCU1_GearCmd/5(output5) -> or5/4
  VCU1_GearCmd/6(output6) -> or6/4
  VCU1_GearCmd/7(output7) -> or7/4
  VCU1_GearCmd/8(output8) -> or8/4
  VCU1_CtrlModel/1(output1) -> or1/5
  VCU1_CtrlModel/2(output2) -> or2/5
  VCU1_CtrlModel/3(output3) -> or3/5
  VCU1_CtrlModel/4(output4) -> or4/5
  VCU1_CtrlModel/5(output5) -> or5/5
  VCU1_CtrlModel/6(output6) -> or6/5
  VCU1_CtrlModel/7(output7) -> or7/5
  VCU1_CtrlModel/8(output8) -> or8/5
  VCU1_EnableReq/1(output1) -> or1/6
  VCU1_EnableReq/2(output2) -> or2/6
  VCU1_EnableReq/3(output3) -> or3/6
  VCU1_EnableReq/4(output4) -> or4/6
  VCU1_EnableReq/5(output5) -> or5/6
  VCU1_EnableReq/6(output6) -> or6/6
  VCU1_EnableReq/7(output7) -> or7/6
  VCU1_EnableReq/8(output8) -> or8/6
  or1/1 -> Conv1/1
  Conv1/1 -> VCU1_mux/1
  or2/1 -> Conv2/1
  Conv2/1 -> VCU1_mux/2
  or3/1 -> Conv3/1
  Conv3/1 -> VCU1_mux/3
  or4/1 -> Conv4/1
  Conv4/1 -> VCU1_mux/4
  or5/1 -> Conv5/1
  Conv5/1 -> VCU1_mux/5
  or6/1 -> Conv6/1
  Conv6/1 -> VCU1_mux/6
  or7/1 -> Conv7/1
  Conv7/1 -> VCU1_mux/7
  or8/1 -> Conv8/1
  Conv8/1 -> VCU1_mux/8
  VCU1_ID/1 -> VCU1_ID_Out/1
  VCU1_DLC/1 -> VCU1_DLC_Out/1
  VCU1_LifeCnt_in/1 -> VCU1_LifeCnt/1(VCU1_LifeCnt)
  VCU1_TorqueRef_in/1 -> VCU1_TorqueRef/1(VCU1_TorqueRef)
  VCU1_SpeedMax_in/1 -> VCU1_SpeedMax/1(VCU1_SpeedMax)
  VCU1_GearCmd_in/1 -> VCU1_GearCmd/1(VCU1_GearCmd)
  VCU1_CtrlModel_in/1 -> VCU1_CtrlModel/1(VCU1_CtrlModel)
  VCU1_EnableReq_in/1 -> VCU1_EnableReq/1(VCU1_EnableReq)

== system six_plus_six_AcmsteeringV09_main_1lf/Subsystem/VCU5 ==
  VCU1_EnableReq_in : Inport
  VCU1_CtrlModel_in : Inport  Port=2
  VCU1_GearCmd_in : Inport  Port=3
  VCU1_SpeedMax_in : Inport  Port=4
  VCU1_TorqueRef_in : Inport  Port=5
  VCU1_LifeCnt_in : Inport  Port=6
  Conv{1..8} (8 alike) : DataTypeConversion
  VCU1_CtrlModel : Subsystem
  VCU1_DLC : Constant  Value=8  OutDataTypeStr=uint8
  VCU1_DLC_Out : Terminator
  VCU1_EnableReq : Subsystem
  VCU1_GearCmd : Subsystem
  VCU1_ID : Constant  Value=2353065767  OutDataTypeStr=single
  VCU1_ID_Out : Terminator
  VCU1_LifeCnt : Subsystem
  VCU1_SpeedMax : Subsystem
  VCU1_TorqueRef : Subsystem
  VCU1_mux : Mux  Inputs=8
  or{1..8} (8 alike) : simulink/Logic and Bit Operations/Bitwise Operator  logicop=OR  UseBitMask=off  NumInputPorts=6  BitMask=bin2dec('11011001')  BitMaskRealWorld=Stored Integer
  output : Outport
  wires:
  VCU1_mux/1 -> output/1
  VCU1_LifeCnt/1(output1) -> or1/1
  VCU1_LifeCnt/2(output2) -> or2/1
  VCU1_LifeCnt/3(output3) -> or3/1
  VCU1_LifeCnt/4(output4) -> or4/1
  VCU1_LifeCnt/5(output5) -> or5/1
  VCU1_LifeCnt/6(output6) -> or6/1
  VCU1_LifeCnt/7(output7) -> or7/1
  VCU1_LifeCnt/8(output8) -> or8/1
  VCU1_TorqueRef/1(output1) -> or1/2
  VCU1_TorqueRef/2(output2) -> or2/2
  VCU1_TorqueRef/3(output3) -> or3/2
  VCU1_TorqueRef/4(output4) -> or4/2
  VCU1_TorqueRef/5(output5) -> or5/2
  VCU1_TorqueRef/6(output6) -> or6/2
  VCU1_TorqueRef/7(output7) -> or7/2
  VCU1_TorqueRef/8(output8) -> or8/2
  VCU1_SpeedMax/1(output1) -> or1/3
  VCU1_SpeedMax/2(output2) -> or2/3
  VCU1_SpeedMax/3(output3) -> or3/3
  VCU1_SpeedMax/4(output4) -> or4/3
  VCU1_SpeedMax/5(output5) -> or5/3
  VCU1_SpeedMax/6(output6) -> or6/3
  VCU1_SpeedMax/7(output7) -> or7/3
  VCU1_SpeedMax/8(output8) -> or8/3
  VCU1_GearCmd/1(output1) -> or1/4
  VCU1_GearCmd/2(output2) -> or2/4
  VCU1_GearCmd/3(output3) -> or3/4
  VCU1_GearCmd/4(output4) -> or4/4
  VCU1_GearCmd/5(output5) -> or5/4
  VCU1_GearCmd/6(output6) -> or6/4
  VCU1_GearCmd/7(output7) -> or7/4
  VCU1_GearCmd/8(output8) -> or8/4
  VCU1_CtrlModel/1(output1) -> or1/5
  VCU1_CtrlModel/2(output2) -> or2/5
  VCU1_CtrlModel/3(output3) -> or3/5
  VCU1_CtrlModel/4(output4) -> or4/5
  VCU1_CtrlModel/5(output5) -> or5/5
  VCU1_CtrlModel/6(output6) -> or6/5
  VCU1_CtrlModel/7(output7) -> or7/5
  VCU1_CtrlModel/8(output8) -> or8/5
  VCU1_EnableReq/1(output1) -> or1/6
  VCU1_EnableReq/2(output2) -> or2/6
  VCU1_EnableReq/3(output3) -> or3/6
  VCU1_EnableReq/4(output4) -> or4/6
  VCU1_EnableReq/5(output5) -> or5/6
  VCU1_EnableReq/6(output6) -> or6/6
  VCU1_EnableReq/7(output7) -> or7/6
  VCU1_EnableReq/8(output8) -> or8/6
  or1/1 -> Conv1/1
  Conv1/1 -> VCU1_mux/1
  or2/1 -> Conv2/1
  Conv2/1 -> VCU1_mux/2
  or3/1 -> Conv3/1
  Conv3/1 -> VCU1_mux/3
  or4/1 -> Conv4/1
  Conv4/1 -> VCU1_mux/4
  or5/1 -> Conv5/1
  Conv5/1 -> VCU1_mux/5
  or6/1 -> Conv6/1
  Conv6/1 -> VCU1_mux/6
  or7/1 -> Conv7/1
  Conv7/1 -> VCU1_mux/7
  or8/1 -> Conv8/1
  Conv8/1 -> VCU1_mux/8
  VCU1_ID/1 -> VCU1_ID_Out/1
  VCU1_DLC/1 -> VCU1_DLC_Out/1
  VCU1_LifeCnt_in/1 -> VCU1_LifeCnt/1(VCU1_LifeCnt)
  VCU1_TorqueRef_in/1 -> VCU1_TorqueRef/1(VCU1_TorqueRef)
  VCU1_SpeedMax_in/1 -> VCU1_SpeedMax/1(VCU1_SpeedMax)
  VCU1_GearCmd_in/1 -> VCU1_GearCmd/1(VCU1_GearCmd)
  VCU1_CtrlModel_in/1 -> VCU1_CtrlModel/1(VCU1_CtrlModel)
  VCU1_EnableReq_in/1 -> VCU1_EnableReq/1(VCU1_EnableReq)

== system six_plus_six_AcmsteeringV09_main_1lf/Subsystem/VCU6 ==
  VCU1_EnableReq_in : Inport
  VCU1_CtrlModel_in : Inport  Port=2
  VCU1_GearCmd_in : Inport  Port=3
  VCU1_SpeedMax_in : Inport  Port=4
  VCU1_TorqueRef_in : Inport  Port=5
  VCU1_LifeCnt_in : Inport  Port=6
  Conv{1..8} (8 alike) : DataTypeConversion
  VCU1_CtrlModel : Subsystem
  VCU1_DLC : Constant  Value=8  OutDataTypeStr=uint8
  VCU1_DLC_Out : Terminator
  VCU1_EnableReq : Subsystem
  VCU1_GearCmd : Subsystem
  VCU1_ID : Constant  Value=2353065767  OutDataTypeStr=single
  VCU1_ID_Out : Terminator
  VCU1_LifeCnt : Subsystem
  VCU1_SpeedMax : Subsystem
  VCU1_TorqueRef : Subsystem
  VCU1_mux : Mux  Inputs=8
  or{1..8} (8 alike) : simulink/Logic and Bit Operations/Bitwise Operator  logicop=OR  UseBitMask=off  NumInputPorts=6  BitMask=bin2dec('11011001')  BitMaskRealWorld=Stored Integer
  output : Outport
  wires:
  VCU1_mux/1 -> output/1
  VCU1_LifeCnt/1(output1) -> or1/1
  VCU1_LifeCnt/2(output2) -> or2/1
  VCU1_LifeCnt/3(output3) -> or3/1
  VCU1_LifeCnt/4(output4) -> or4/1
  VCU1_LifeCnt/5(output5) -> or5/1
  VCU1_LifeCnt/6(output6) -> or6/1
  VCU1_LifeCnt/7(output7) -> or7/1
  VCU1_LifeCnt/8(output8) -> or8/1
  VCU1_TorqueRef/1(output1) -> or1/2
  VCU1_TorqueRef/2(output2) -> or2/2
  VCU1_TorqueRef/3(output3) -> or3/2
  VCU1_TorqueRef/4(output4) -> or4/2
  VCU1_TorqueRef/5(output5) -> or5/2
  VCU1_TorqueRef/6(output6) -> or6/2
  VCU1_TorqueRef/7(output7) -> or7/2
  VCU1_TorqueRef/8(output8) -> or8/2
  VCU1_SpeedMax/1(output1) -> or1/3
  VCU1_SpeedMax/2(output2) -> or2/3
  VCU1_SpeedMax/3(output3) -> or3/3
  VCU1_SpeedMax/4(output4) -> or4/3
  VCU1_SpeedMax/5(output5) -> or5/3
  VCU1_SpeedMax/6(output6) -> or6/3
  VCU1_SpeedMax/7(output7) -> or7/3
  VCU1_SpeedMax/8(output8) -> or8/3
  VCU1_GearCmd/1(output1) -> or1/4
  VCU1_GearCmd/2(output2) -> or2/4
  VCU1_GearCmd/3(output3) -> or3/4
  VCU1_GearCmd/4(output4) -> or4/4
  VCU1_GearCmd/5(output5) -> or5/4
  VCU1_GearCmd/6(output6) -> or6/4
  VCU1_GearCmd/7(output7) -> or7/4
  VCU1_GearCmd/8(output8) -> or8/4
  VCU1_CtrlModel/1(output1) -> or1/5
  VCU1_CtrlModel/2(output2) -> or2/5
  VCU1_CtrlModel/3(output3) -> or3/5
  VCU1_CtrlModel/4(output4) -> or4/5
  VCU1_CtrlModel/5(output5) -> or5/5
  VCU1_CtrlModel/6(output6) -> or6/5
  VCU1_CtrlModel/7(output7) -> or7/5
  VCU1_CtrlModel/8(output8) -> or8/5
  VCU1_EnableReq/1(output1) -> or1/6
  VCU1_EnableReq/2(output2) -> or2/6
  VCU1_EnableReq/3(output3) -> or3/6
  VCU1_EnableReq/4(output4) -> or4/6
  VCU1_EnableReq/5(output5) -> or5/6
  VCU1_EnableReq/6(output6) -> or6/6
  VCU1_EnableReq/7(output7) -> or7/6
  VCU1_EnableReq/8(output8) -> or8/6
  or1/1 -> Conv1/1
  Conv1/1 -> VCU1_mux/1
  or2/1 -> Conv2/1
  Conv2/1 -> VCU1_mux/2
  or3/1 -> Conv3/1
  Conv3/1 -> VCU1_mux/3
  or4/1 -> Conv4/1
  Conv4/1 -> VCU1_mux/4
  or5/1 -> Conv5/1
  Conv5/1 -> VCU1_mux/5
  or6/1 -> Conv6/1
  Conv6/1 -> VCU1_mux/6
  or7/1 -> Conv7/1
  Conv7/1 -> VCU1_mux/7
  or8/1 -> Conv8/1
  Conv8/1 -> VCU1_mux/8
  VCU1_ID/1 -> VCU1_ID_Out/1
  VCU1_DLC/1 -> VCU1_DLC_Out/1
  VCU1_LifeCnt_in/1 -> VCU1_LifeCnt/1(VCU1_LifeCnt)
  VCU1_TorqueRef_in/1 -> VCU1_TorqueRef/1(VCU1_TorqueRef)
  VCU1_SpeedMax_in/1 -> VCU1_SpeedMax/1(VCU1_SpeedMax)
  VCU1_GearCmd_in/1 -> VCU1_GearCmd/1(VCU1_GearCmd)
  VCU1_CtrlModel_in/1 -> VCU1_CtrlModel/1(VCU1_CtrlModel)
  VCU1_EnableReq_in/1 -> VCU1_EnableReq/1(VCU1_EnableReq)

== system six_plus_six_AcmsteeringV09_main_1lf/Data_input/1/Enabled Subsystem ==
  In2 : Inport
  Enable : EnablePort
  Add : Sum
  Constant : Constant  Value=256
  Constant1 : Constant  SampleTime=-1
  Constant3 : Constant  Value=256
  Data Type Conversion{8..13} (6 alike) : DataTypeConversion  OutDataTypeStr=uint8
  Demux1 : Demux  Outputs=6
  MATLAB Function1 : MATLAB Function  TreatAsAtomicUnit=on
  MATLAB Function3 : MATLAB Function  TreatAsAtomicUnit=on
  Memory : Memory  InheritSampleTime=on
  Product : Product
  Product2 : Product
  Saturation : Saturate  UpperLimit=5  LowerLimit=0
  Sum : Sum  Inputs=|++
  Sum1 : Sum  Inputs=|++
  Terminator1 : Terminator
  Terminator2 : Terminator
  motec_spd_2 : Outport
  motec_current_2 : Outport  Port=2
  enable_count2 : Outport  Port=3
  wires:
  In2/1 -> Demux1/1
  Demux1/1 -> Data Type Conversion8/1
  Demux1/2 -> Data Type Conversion9/1
  Demux1/3 -> Data Type Conversion10/1
  Demux1/4 -> Data Type Conversion11/1
  Demux1/5 -> Data Type Conversion13/1
  Demux1/6 -> Data Type Conversion12/1
  Data Type Conversion8/1 -> Terminator1/1
  Data Type Conversion9/1 -> Terminator2/1
  Data Type Conversion10/1 -> Sum/1
  Data Type Conversion11/1 -> Product/2
  Constant/1 -> Product/1
  Product/1 -> Sum/2
  Sum/1 -> MATLAB Function3/1(speed)
  Data Type Conversion12/1 -> Product2/2
  Constant3/1 -> Product2/1
  Product2/1 -> Sum1/2
  Data Type Conversion13/1 -> Sum1/1
  Sum1/1 -> MATLAB Function1/1(current_in)
  MATLAB Function3/1(speed_out) -> motec_spd_2/1
  MATLAB Function1/1(current_out) -> motec_current_2/1
  Constant1/1 -> Add/1
  Memory/1 -> Add/2
  Add/1 -> Saturation/1
  Saturation/1 -> enable_count2/1, Memory/1

== system six_plus_six_AcmsteeringV09_main_1lf/Data_input/10/Enabled Subsystem ==
  In2 : Inport
  Enable : EnablePort
  Data Type Conversion{,1..7} (8 alike) : DataTypeConversion
  Demux1 : Demux  Outputs=8
  MATLAB Function : MATLAB Function  TreatAsAtomicUnit=on
  MATLAB Function1 : MATLAB Function  TreatAsAtomicUnit=on
  Rolling_Out : Outport
  Heading_Out : Outport  Port=2
  wires:
  Demux1/8 -> Data Type Conversion3/1
  Demux1/7 -> Data Type Conversion2/1
  Demux1/6 -> Data Type Conversion1/1
  Demux1/5 -> Data Type Conversion/1
  MATLAB Function1/1(y) -> Heading_Out/1
  MATLAB Function/1(y) -> Rolling_Out/1
  Demux1/1 -> Data Type Conversion4/1
  Demux1/2 -> Data Type Conversion5/1
  Demux1/3 -> Data Type Conversion6/1
  Demux1/4 -> Data Type Conversion7/1
  In2/1 -> Demux1/1
  Data Type Conversion/1 -> MATLAB Function1/1(data1)
  Data Type Conversion1/1 -> MATLAB Function1/2(data2)
  Data Type Conversion2/1 -> MATLAB Function1/3(data3)
  Data Type Conversion3/1 -> MATLAB Function1/4(data4)
  Data Type Conversion4/1 -> MATLAB Function/1(data1)
  Data Type Conversion5/1 -> MATLAB Function/2(data2)
  Data Type Conversion6/1 -> MATLAB Function/3(data3)
  Data Type Conversion7/1 -> MATLAB Function/4(data4)

== system six_plus_six_AcmsteeringV09_main_1lf/Data_input/11/Enabled Subsystem ==
  In2 : Inport
  Enable : EnablePort
  Data Type Conversion{,1..7} (8 alike) : DataTypeConversion
  Demux1 : Demux  Outputs=8
  MATLAB Function : MATLAB Function  TreatAsAtomicUnit=on
  Terminator{,1..3} (4 alike) : Terminator
  Pitching_Out : Outport
  wires:
  In2/1 -> Demux1/1
  Demux1/4 -> Data Type Conversion3/1
  Demux1/3 -> Data Type Conversion2/1
  Demux1/2 -> Data Type Conversion1/1
  Demux1/1 -> Data Type Conversion/1
  MATLAB Function/1(y) -> Pitching_Out/1
  Demux1/6 -> Data Type Conversion5/1
  Demux1/5 -> Data Type Conversion4/1
  Demux1/7 -> Data Type Conversion6/1
  Demux1/8 -> Data Type Conversion7/1
  Data Type Conversion/1 -> MATLAB Function/1(data1)
  Data Type Conversion6/1 -> Terminator2/1
  Data Type Conversion3/1 -> MATLAB Function/4(data4)
  Data Type Conversion4/1 -> Terminator/1
  Data Type Conversion7/1 -> Terminator3/1
  Data Type Conversion1/1 -> MATLAB Function/2(data2)
  Data Type Conversion2/1 -> MATLAB Function/3(data3)
  Data Type Conversion5/1 -> Terminator1/1

== system six_plus_six_AcmsteeringV09_main_1lf/Data_input/181/Enabled Subsystem ==
  In2 : Inport
  Enable : EnablePort
  Add : Sum
  Constant : Constant  Value=256
  Constant1 : Constant  SampleTime=-1
  Constant3 : Constant  Value=256
  Data Type Conversion{8..13} (6 alike) : DataTypeConversion  OutDataTypeStr=uint8
  Demux1 : Demux  Outputs=6
  MATLAB Function1 : MATLAB Function  TreatAsAtomicUnit=on
  MATLAB Function3 : MATLAB Function  TreatAsAtomicUnit=on
  Memory : Memory  InheritSampleTime=on
  Product : Product
  Product2 : Product
  Saturation : Saturate  UpperLimit=5  LowerLimit=0
  Sum : Sum  Inputs=|++
  Sum1 : Sum  Inputs=|++
  Terminator1 : Terminator
  Terminator2 : Terminator
  motec_spd_1 : Outport
  motec_current_1 : Outport  Port=2
  enable_count1 : Outport  Port=3
  wires:
  In2/1 -> Demux1/1
  Demux1/1 -> Data Type Conversion8/1
  Demux1/2 -> Data Type Conversion9/1
  Demux1/3 -> Data Type Conversion10/1
  Demux1/4 -> Data Type Conversion11/1
  Demux1/5 -> Data Type Conversion13/1
  Demux1/6 -> Data Type Conversion12/1
  Data Type Conversion8/1 -> Terminator1/1
  Data Type Conversion9/1 -> Terminator2/1
  Data Type Conversion10/1 -> Sum/1
  Data Type Conversion11/1 -> Product/2
  Constant/1 -> Product/1
  Product/1 -> Sum/2
  Sum/1 -> MATLAB Function3/1(speed)
  Data Type Conversion12/1 -> Product2/2
  Constant3/1 -> Product2/1
  Product2/1 -> Sum1/2
  Data Type Conversion13/1 -> Sum1/1
  Sum1/1 -> MATLAB Function1/1(current_in)
  MATLAB Function3/1(speed_out) -> motec_spd_1/1
  MATLAB Function1/1(current_out) -> motec_current_1/1
  Constant1/1 -> Add/1
  Memory/1 -> Add/2
  Add/1 -> Saturation/1
  Saturation/1 -> enable_count1/1, Memory/1

== system six_plus_six_AcmsteeringV09_main_1lf/Data_input/2/Enabled Subsystem ==
  In2 : Inport
  Enable : EnablePort
  Add : Sum
  Constant : Constant  Value=256
  Constant1 : Constant  SampleTime=-1
  Constant3 : Constant  Value=256
  Data Type Conversion{8..13} (6 alike) : DataTypeConversion  OutDataTypeStr=uint8
  Demux1 : Demux  Outputs=6
  MATLAB Function1 : MATLAB Function  TreatAsAtomicUnit=on
  MATLAB Function3 : MATLAB Function  TreatAsAtomicUnit=on
  Memory : Memory  InheritSampleTime=on
  Product : Product
  Product2 : Product
  Saturation : Saturate  UpperLimit=5  LowerLimit=0
  Sum : Sum  Inputs=|++
  Sum1 : Sum  Inputs=|++
  Terminator1 : Terminator
  Terminator2 : Terminator
  motec_spd_4 : Outport
  motec_current_4 : Outport  Port=2
  enable_count1 : Outport  Port=3
  wires:
  MATLAB Function1/1(current_out) -> motec_current_4/1
  MATLAB Function3/1(speed_out) -> motec_spd_4/1
  Sum1/1 -> MATLAB Function1/1(current_in)
  Data Type Conversion13/1 -> Sum1/1
  Product2/1 -> Sum1/2
  Constant3/1 -> Product2/1
  Data Type Conversion12/1 -> Product2/2
  Sum/1 -> MATLAB Function3/1(speed)
  Product/1 -> Sum/2
  Constant/1 -> Product/1
  Data Type Conversion11/1 -> Product/2
  Data Type Conversion10/1 -> Sum/1
  Data Type Conversion9/1 -> Terminator2/1
  Data Type Conversion8/1 -> Terminator1/1
  Demux1/6 -> Data Type Conversion12/1
  Demux1/5 -> Data Type Conversion13/1
  Demux1/4 -> Data Type Conversion11/1
  Demux1/3 -> Data Type Conversion10/1
  Demux1/2 -> Data Type Conversion9/1
  Demux1/1 -> Data Type Conversion8/1
  In2/1 -> Demux1/1
  Constant1/1 -> Add/1
  Memory/1 -> Add/2
  Add/1 -> Saturation/1
  Saturation/1 -> enable_count1/1, Memory/1

== system six_plus_six_AcmsteeringV09_main_1lf/Data_input/3/Enabled Subsystem ==
  In2 : Inport
  Enable : EnablePort
  Add : Sum
  Constant : Constant  Value=256
  Constant1 : Constant  SampleTime=-1
  Constant3 : Constant  Value=256
  Data Type Conversion{8..13} (6 alike) : DataTypeConversion  OutDataTypeStr=uint8
  Demux1 : Demux  Outputs=6
  MATLAB Function1 : MATLAB Function  TreatAsAtomicUnit=on
  MATLAB Function3 : MATLAB Function  TreatAsAtomicUnit=on
  Memory : Memory  InheritSampleTime=on
  Product : Product
  Product2 : Product
  Saturation : Saturate  UpperLimit=5  LowerLimit=0
  Sum : Sum  Inputs=|++
  Sum1 : Sum  Inputs=|++
  Terminator1 : Terminator
  Terminator2 : Terminator
  motec_spd_3 : Outport
  motec_current_3 : Outport  Port=2
  enable_count1 : Outport  Port=3
  wires:
  MATLAB Function1/1(current_out) -> motec_current_3/1
  MATLAB Function3/1(speed_out) -> motec_spd_3/1
  Sum1/1 -> MATLAB Function1/1(current_in)
  Data Type Conversion13/1 -> Sum1/1
  Product2/1 -> Sum1/2
  Constant3/1 -> Product2/1
  Data Type Conversion12/1 -> Product2/2
  Sum/1 -> MATLAB Function3/1(speed)
  Product/1 -> Sum/2
  Constant/1 -> Product/1
  Data Type Conversion11/1 -> Product/2
  Data Type Conversion10/1 -> Sum/1
  Data Type Conversion9/1 -> Terminator2/1
  Data Type Conversion8/1 -> Terminator1/1
  Demux1/6 -> Data Type Conversion12/1
  Demux1/5 -> Data Type Conversion13/1
  Demux1/4 -> Data Type Conversion11/1
  Demux1/3 -> Data Type Conversion10/1
  Demux1/2 -> Data Type Conversion9/1
  Demux1/1 -> Data Type Conversion8/1
  In2/1 -> Demux1/1
  Constant1/1 -> Add/1
  Memory/1 -> Add/2
  Add/1 -> Saturation/1
  Saturation/1 -> enable_count1/1, Memory/1

== system six_plus_six_AcmsteeringV09_main_1lf/Data_input/4/Enabled Subsystem ==
  In2 : Inport
  Enable : EnablePort
  Data Type Conversion{,1..7} (8 alike) : DataTypeConversion
  Demux1 : Demux  Outputs=8
  MATLAB Function : MATLAB Function  TreatAsAtomicUnit=on
  MATLAB Function1 : MATLAB Function  TreatAsAtomicUnit=on
  Xangularrate_Out : Outport
  Yangularrate_Out : Outport  Port=2
  wires:
  In2/1 -> Demux1/1
  Demux1/4 -> Data Type Conversion3/1
  Demux1/3 -> Data Type Conversion2/1
  Demux1/2 -> Data Type Conversion1/1
  Demux1/1 -> Data Type Conversion/1
  MATLAB Function/1(y) -> Xangularrate_Out/1
  MATLAB Function1/1(y) -> Yangularrate_Out/1
  Demux1/5 -> Data Type Conversion4/1
  Demux1/6 -> Data Type Conversion5/1
  Demux1/7 -> Data Type Conversion6/1
  Demux1/8 -> Data Type Conversion7/1
  Data Type Conversion/1 -> MATLAB Function/1(data1)
  Data Type Conversion1/1 -> MATLAB Function/2(data2)
  Data Type Conversion2/1 -> MATLAB Function/3(data3)
  Data Type Conversion3/1 -> MATLAB Function/4(data4)
  Data Type Conversion4/1 -> MATLAB Function1/1(data1)
  Data Type Conversion5/1 -> MATLAB Function1/2(data2)
  Data Type Conversion6/1 -> MATLAB Function1/3(data3)
  Data Type Conversion7/1 -> MATLAB Function1/4(data4)
